simulink model "CoVMD_TrqLeadCoord"  (R2016b)
settings: configuration reference "CodeGenConfigSet" (kept outside this file)
undefined symbols (not defined in the file or in its folder): Switch_conv, WESDem_State_conv
libraries: simulink x1
settings Model: Creator=Colin  LastModifiedBy=liutao
settings ConfigSetRef: SourceLocation=Base Workspace

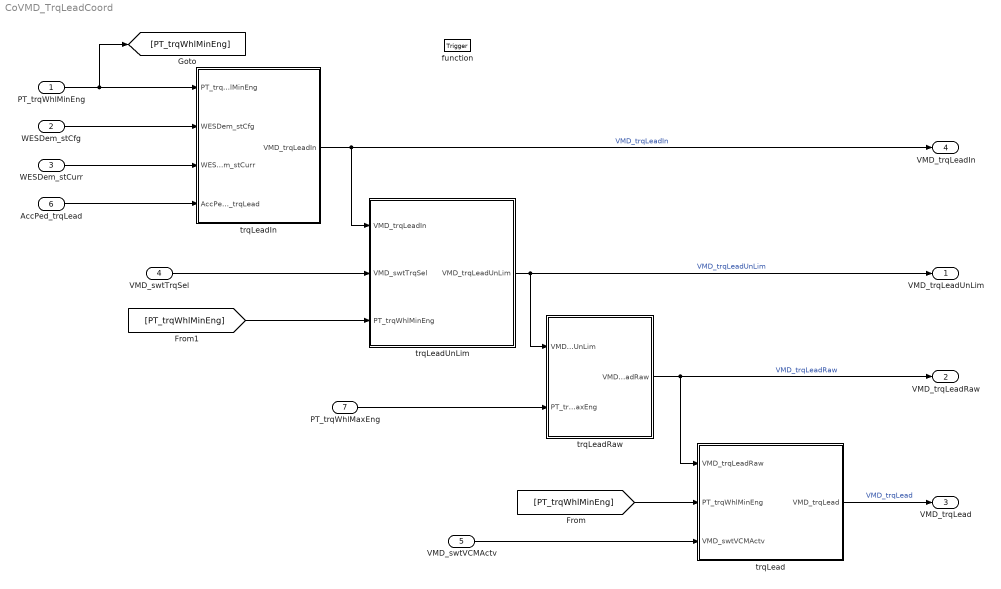
== system CoVMD_TrqLeadCoord ==
  PT_trqWhlMinEng : Inport  Tag=Nm  Description=Minimum wheel torque from the engine  OutMin=-3000  OutMax=3000  OutDataTypeStr=Trq_Nm
  WESDem_stCfg : Inport  Description=Configuration of the actual operating mode  Port=2  OutMin=0  OutMax=65535  OutDataTypeStr=State_uint16
  WESDem_stCurr : Inport  Description=Status of the working engine Speed Control  Port=3  OutDataTypeStr=Enum: WESDem_State_conv
  VMD_swtTrqSel : Inport  Description=Driver demand - Cruise control torque selection switch  Port=4  OutMin=0  OutMax=255  OutDataTypeStr=State_uint8
  VMD_swtVCMActv : Inport  Description=Application parameter which Indicates whether Vehicle Control Mode(VCM) is enabled or disabled  Port=5  OutDataTypeStr=Enum: Switch_conv
  AccPed_trqLead : Inport  Tag=Nm  Description=Lead torque of accelerator pedal  Port=6  OutMin=-3000  OutMax=3000  OutDataTypeStr=Trq_Nm
  PT_trqWhlMaxEng : Inport  Tag=Nm  Description=Maximum wheel torque from the engine  Port=7  OutMin=-3000  OutMax=3000  OutDataTypeStr=Trq_Nm
  function : TriggerPort  TriggerType=function-call  VariantControl=Variant
  trqLead : Subsystem
  trqLeadIn : Subsystem
  trqLeadRaw : Subsystem
  trqLeadUnLim : Subsystem
  VMD_trqLeadUnLim : Outport  Tag=Nm  Description=Unlimited propulsion lead torque.  OutMin=-3000  OutMax=3000  OutDataTypeStr=Trq_Nm
  VMD_trqLeadRaw : Outport  Tag=Nm  Description=Raw value of propulsion lead torque after driving assistance coordination  Port=2  OutMin=-3000  OutMax=3000  OutDataTypeStr=Trq_Nm
  VMD_trqLead : Outport  Tag=Nm  Description=propulsion lead torque after driving assistance coordination  Port=3  OutMin=-3000  OutMax=3000  OutDataTypeStr=Trq_Nm
  VMD_trqLeadIn : Outport  Tag=Nm  Description=lead torque of Propulsion and Brake  Port=4  OutMin=-3000  OutMax=3000  OutDataTypeStr=Trq_Nm
  wires:
  trqLeadUnLim/1(VMD_trqLeadUnLim) -> trqLeadRaw/1(VMD_trqLeadUnLim), VMD_trqLeadUnLim/1  "VMD_trqLeadUnLim"
  trqLeadRaw/1(VMD_trqLeadRaw) -> trqLead/1(VMD_trqLeadRaw), VMD_trqLeadRaw/1  "VMD_trqLeadRaw"
  trqLead/1(VMD_trqLead) -> VMD_trqLead/1  "VMD_trqLead"
  trqLeadIn/1(VMD_trqLeadIn) -> trqLeadUnLim/1(VMD_trqLeadIn), VMD_trqLeadIn/1  "VMD_trqLeadIn"
  PT_trqWhlMinEng/1 -> [PT_trqWhlMinEng], trqLeadIn/1(PT_trqWhlMinEng)
  WESDem_stCfg/1 -> trqLeadIn/2(WESDem_stCfg)
  WESDem_stCurr/1 -> trqLeadIn/3(WESDem_stCurr)
  AccPed_trqLead/1 -> trqLeadIn/4(AccPed_trqLead)
  VMD_swtTrqSel/1 -> trqLeadUnLim/2(VMD_swtTrqSel)
  PT_trqWhlMaxEng/1 -> trqLeadRaw/2(PT_trqWhlMaxEng)
  [PT_trqWhlMinEng] -> trqLead/2(PT_trqWhlMinEng)
  VMD_swtVCMActv/1 -> trqLead/3(VMD_swtVCMActv)
  [PT_trqWhlMinEng] -> trqLeadUnLim/3(PT_trqWhlMinEng)

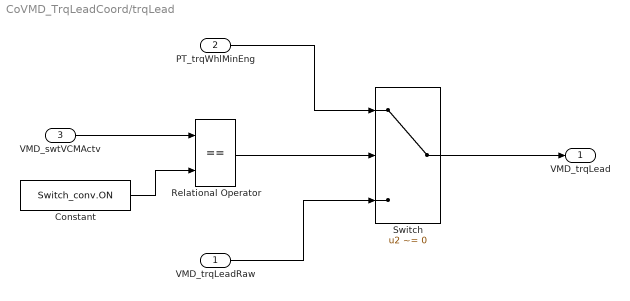
== system CoVMD_TrqLeadCoord/trqLead ==
  VMD_trqLeadRaw : Inport
  PT_trqWhlMinEng : Inport  Port=2
  VMD_swtVCMActv : Inport  Port=3
  Constant : Constant  Value=Switch_conv.ON
  Relational Operator : RelationalOperator  Operator===  OutDataTypeStr=boolean  RndMeth=Simplest
  Switch : Switch  Criteria=u2 ~= 0
  VMD_trqLead : Outport
  wires:
  VMD_swtVCMActv/1 -> Relational Operator/1
  Constant/1 -> Relational Operator/2
  Relational Operator/1 -> Switch/2
  VMD_trqLeadRaw/1 -> Switch/3
  PT_trqWhlMinEng/1 -> Switch/1
  Switch/1 -> VMD_trqLead/1

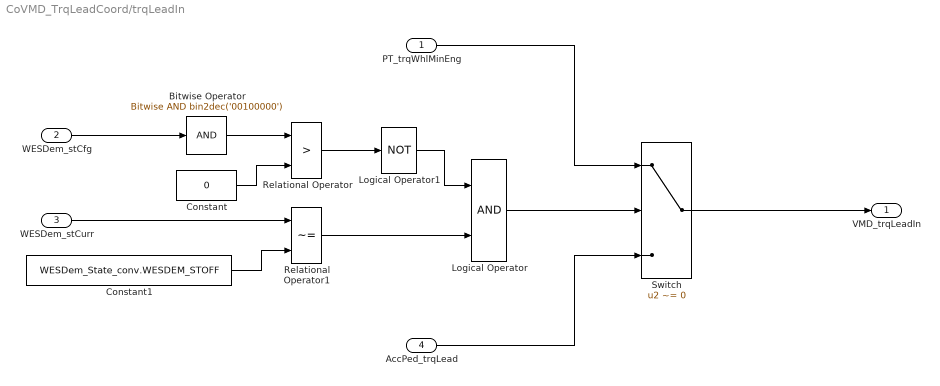
== system CoVMD_TrqLeadCoord/trqLeadIn ==
  PT_trqWhlMinEng : Inport
  WESDem_stCfg : Inport  Port=2
  WESDem_stCurr : Inport  Port=3
  AccPed_trqLead : Inport  Port=4
  Bitwise Operator : simulink/Logic and Bit Operations/Bitwise Operator  logicop=AND  UseBitMask=on  BitMask=bin2dec('00100000')  BitMaskRealWorld=Stored Integer
  Constant : Constant  Value=0  OutDataTypeStr=Inherit: Inherit via back propagation
  Constant1 : Constant  Value=WESDem_State_conv.WESDEM_STOFF
  Logical Operator : Logic  AllPortsSameDT=off  OutDataTypeStr=boolean
  Logical Operator1 : Logic  Operator=NOT  AllPortsSameDT=off  OutDataTypeStr=boolean
  Relational Operator : RelationalOperator  Operator=>  OutDataTypeStr=boolean  RndMeth=Simplest  InputSameDT=on
  Relational Operator1 : RelationalOperator  Operator=~=  OutDataTypeStr=boolean  RndMeth=Simplest
  Switch : Switch  Criteria=u2 ~= 0
  VMD_trqLeadIn : Outport
  wires:
  WESDem_stCfg/1 -> Bitwise Operator/1
  Bitwise Operator/1 -> Relational Operator/1
  Constant/1 -> Relational Operator/2
  Relational Operator/1 -> Logical Operator1/1
  Logical Operator1/1 -> Logical Operator/1
  Relational Operator1/1 -> Logical Operator/2
  WESDem_stCurr/1 -> Relational Operator1/1
  Constant1/1 -> Relational Operator1/2
  Logical Operator/1 -> Switch/2
  PT_trqWhlMinEng/1 -> Switch/1
  AccPed_trqLead/1 -> Switch/3
  Switch/1 -> VMD_trqLeadIn/1

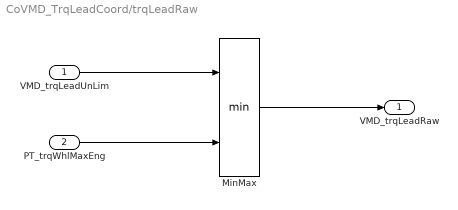
== system CoVMD_TrqLeadCoord/trqLeadRaw ==
  VMD_trqLeadUnLim : Inport
  PT_trqWhlMaxEng : Inport  Port=2
  MinMax : MinMax  Inputs=2
  VMD_trqLeadRaw : Outport
  wires:
  VMD_trqLeadUnLim/1 -> MinMax/1
  PT_trqWhlMaxEng/1 -> MinMax/2
  MinMax/1 -> VMD_trqLeadRaw/1

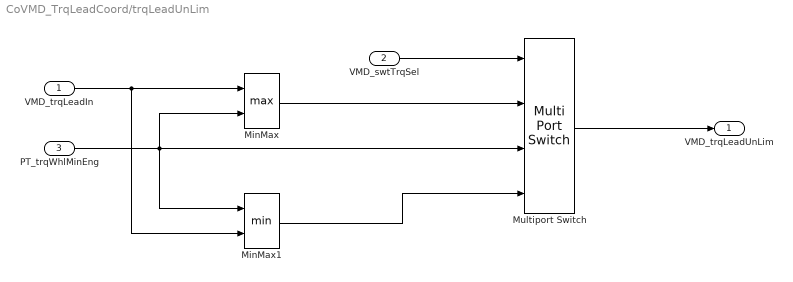
== system CoVMD_TrqLeadCoord/trqLeadUnLim ==
  VMD_trqLeadIn : Inport
  VMD_swtTrqSel : Inport  Port=2
  PT_trqWhlMinEng : Inport  Port=3
  MinMax : MinMax  Function=max  Inputs=2
  MinMax1 : MinMax  Inputs=2
  Multiport Switch : MultiPortSwitch  DataPortOrder=Specify indices  DataPortIndices={1,2,10}
  VMD_trqLeadUnLim : Outport
  wires:
  VMD_swtTrqSel/1 -> Multiport Switch/1
  Multiport Switch/1 -> VMD_trqLeadUnLim/1
  VMD_trqLeadIn/1 -> MinMax1/2, MinMax/1
  PT_trqWhlMinEng/1 -> MinMax1/1, MinMax/2, Multiport Switch/3
  MinMax/1 -> Multiport Switch/2
  MinMax1/1 -> Multiport Switch/4
